simulink model "model_simulink"  (R2017a)
settings: Solver=VariableStepAuto  StartTime=0.0  StopTime=0.02  RelTol=1e-3
libraries: dsparch4 x1
settings Model: Creator=root  LastModifiedBy=root

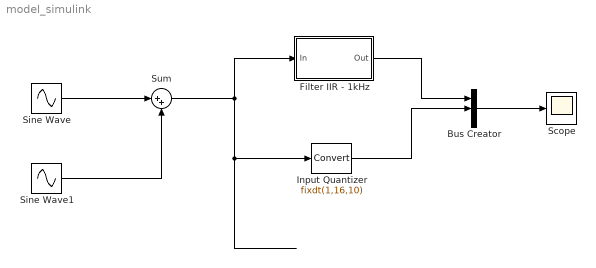
== system model_simulink ==
  Bus Creator : BusCreator  Inputs=3
  Filter IIR - 1kHz : Subsystem  Tag=BlockMethodSubSystem
  Input Quantizer : DataTypeConversion  OutDataTypeStr=fixdt(1,16,10)  RndMeth=Round  SaturateOnIntegerOverflow=on
  Scope : Scope
  Sine Wave : Sin  Frequency=2*pi*500  SampleTime=0
  Sine Wave1 : Sin  Frequency=2*pi*15000  SampleTime=0
  Sum : Sum  Inputs=|++
  wires:
  Bus Creator/1 -> Scope/1
  Sine Wave/1 -> Sum/1
  Sine Wave1/1 -> Sum/2
  Sum/1 -> Input Quantizer/1, Filter IIR - 1kHz/1(In)
  Filter IIR - 1kHz/1(Out) -> Bus Creator/1
  Input Quantizer/1 -> Bus Creator/2

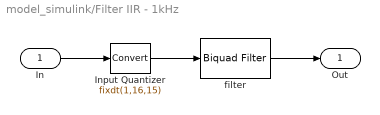
== system model_simulink/Filter IIR - 1kHz ==
  In : Inport
  Input Quantizer : DataTypeConversion  OutDataTypeStr=fixdt(1,16,15)  RndMeth=Round  SaturateOnIntegerOverflow=on
  filter : dsparch4/Biquad Filter  IIRFiltStruct=Direct form II  CoeffSource=Specify via dialog  BiQuadCoeffs=[1 2 1 1 -1.90553352732601722 0.926549887892354818;1 2 1 1 -1.79157222204845579 0.811331689546275991;1 2 1 1 -1.73177624438811617 0.750876214790290986]  a0Flag=Warning  IC=0  ICnum=0  ICden=0  InputProcessing=Columns as channels (frame based)  firstCoeffMode=Binary point scaling  firstCoeffWordLength=16  firstCoeffFracLength=13  outputMode=Binary point scaling  outputWordLength=16  outputFracLength=10  accumMode=Binary point scaling  accumWordLength=40  accumFracLength=28  denAccumFracLength=29  prodOutputMode=Binary point scaling  prodOutputWordLength=32  prodOutputFracLength=28  denProdOutputFracLength=29  memoryMode=Binary point scaling  memoryWordLength=16  memoryFracLength=15  secondMemoryFracLength=15  roundingMode=Convergent  overflowMode=off  ScaleValues=[0.00525409014158444588;0.00493986687445507801;0.00477499260054373587;1]  optimizeScaleValues=on  ScaleValueMode=Specify via input port (g)  scaleValueFracLength=22  stageInputMode=Binary point scaling  stageOutputMode=Binary point scaling  stageInputWordLength=16  stageInputFracLength=16  stageOutputWordLength=16  stageOutputFracLength=10  FilterSource=Specify via dialog  FilterObject=BQF
      settings: SourceProductName=DSP System Toolbox
  Out : Outport
  wires:
  In/1 -> Input Quantizer/1
  Input Quantizer/1 -> filter/1
  filter/1 -> Out/1
